simulink model "uav-pid"  (R2020a)
settings: Solver=ode4  StartTime=0.0  StopTime=100  FixedStep=0.25  RelTol=1e-3
libraries: simulink x6
settings Model: Creator=baron  LastModifiedBy=baron

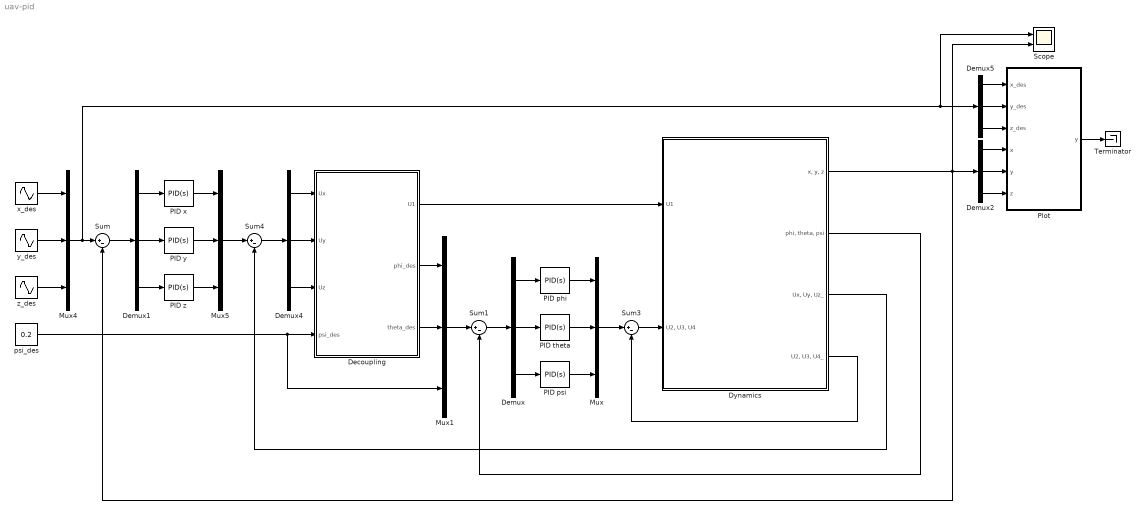
== system uav-pid ==
  Decoupling : MATLAB Function  TreatAsAtomicUnit=on
  Demux{,1..2,4..5} (5 alike) : Demux  Outputs=3
  Dynamics : Subsystem
  Mux{,1,4..5} (4 alike) : Mux  Inputs=3
  PID phi : simulink/Continuous/PID Controller  Controller=PID  Form=Parallel  TimeDomain=Continuous-time  UseExternalTs=off  SampleTime=-1  IntegratorMethod=Forward Euler  FilterMethod=Forward Euler  ControllerParametersSource=internal  P=0.00360663400977862  I=0.000168843771504077  D=0.0189174411465633  UseFilter=on  N=5.45397025421619  TunerSelectOption=Transfer Function Based (PID Tuner App)  InitialConditionSource=internal  InitialConditionForIntegrator=0  InitialConditionForFilter=0  DifferentiatorICPrevScaledInput=0  ExternalReset=none  TrackingMode=off  Kt=1  LimitOutput=off  UpperSaturationLimit=inf  LowerSaturationLimit=-inf  LinearizeAsGain=on  AntiWindupMode=none  Kb=1  POutMin=[]  POutMax=[]  IOutMin=[]  IOutMax=[]  DOutMin=[]  DOutMax=[]  NOutMin=[]  NOutMax=[]  SumOutMin=[]  SumOutMax=[]  SaturationOutMin=[]  SaturationOutMax=[]  PParamMin=[]  PParamMax=[]  IParamMin=[]  IParamMax=[]  DParamMin=[]  DParamMax=[]  NParamMin=[]  NParamMax=[]  KbParamMin=[]  KbParamMax=[]  KtParamMin=[]  KtParamMax=[]  KbOutMin=[]  KbOutMax=[]  KtOutMin=[]  KtOutMax=[]  IntegratorOutMin=[]  IntegratorOutMax=[]  FilterOutMin=[]  FilterOutMax=[]  SumI1OutMin=[]  SumI1OutMax=[]  SumI2OutMin=[]  SumI2OutMax=[]  SumI3OutMin=[]  SumI3OutMax=[]  SumI4OutMin=[]  SumI4OutMax=[]  SumDOutMin=[]  SumDOutMax=[]  DifferentiatorOutMin=[]  DifferentiatorOutMax=[]  FilterDiffOutCoefMin=[]  FilterDiffOutCoefMax=[]  ReciprocalOutMin=[]  ReciprocalOutMax=[]  SumDenOutMin=[]  SumDenOutMax=[]  SumNumOutMin=[]  SumNumOutMax=[]  DivideOutMin=[]  DivideOutMax=[]  UdiffTsProdOutMin=[]  UdiffTsProdOutMax=[]  NTsProdOutMin=[]  NTsProdOutMax=[]  UintegralTsProdOutMin=[]  UintegralTsProdOutMax=[]  UngainTsProdOutMin=[]  UngainTsProdOutMax=[]  IntegratorContinuousStateAttributes=''  IntegratorStateMustResolveToSignalObject=off  IntegratorRTWStateStorageClass=Auto  FilterContinuousStateAttributes=''  FilterStateMustResolveToSignalObject=off  FilterRTWStateStorageClass=Auto  ParallelPVariant=InternalParameters  IdealPVariant=Disabled  IVariant=InternalParameters  DVariant=InternalParameters  IntegratorVariant=Continuous  SatVariant=Disabled  AWVariant=Passthrough  PCopyVariant=Disabled  TRVariant=Disabled  FdbkBlocksVariant=Forward  IdealPFdbkVariant=Disabled  SatFdbkVariant=Disabled  DerivativeFilterVariant=ContFilter  NVariant=InternalParameters  NCopyVariant=Disabled  FilterICVariant=InternalICsFilter  IntegratorICVariant=InternalICs  ExternalResetVariant=Disabled  TRSumVariant=Passthrough  SumFdbkVariant=Disabled  SumVariant=Sum_PID  TsampFilterVariant=InternalTs  TsampNgainVariant=Passthrough  TsampIntegralVariant=Passthrough
  PID psi : simulink/Continuous/PID Controller  Controller=PID  Form=Parallel  TimeDomain=Continuous-time  UseExternalTs=off  SampleTime=-1  IntegratorMethod=Forward Euler  FilterMethod=Forward Euler  ControllerParametersSource=internal  P=0.0016341631960493  I=7.65029876960143e-05  D=0.00857147855904571  UseFilter=on  N=5.45397025421619  TunerSelectOption=Transfer Function Based (PID Tuner App)  InitialConditionSource=internal  InitialConditionForIntegrator=0  InitialConditionForFilter=0  DifferentiatorICPrevScaledInput=0  ExternalReset=none  TrackingMode=off  Kt=1  LimitOutput=off  UpperSaturationLimit=inf  LowerSaturationLimit=-inf  LinearizeAsGain=on  AntiWindupMode=none  Kb=1  POutMin=[]  POutMax=[]  IOutMin=[]  IOutMax=[]  DOutMin=[]  DOutMax=[]  NOutMin=[]  NOutMax=[]  SumOutMin=[]  SumOutMax=[]  SaturationOutMin=[]  SaturationOutMax=[]  PParamMin=[]  PParamMax=[]  IParamMin=[]  IParamMax=[]  DParamMin=[]  DParamMax=[]  NParamMin=[]  NParamMax=[]  KbParamMin=[]  KbParamMax=[]  KtParamMin=[]  KtParamMax=[]  KbOutMin=[]  KbOutMax=[]  KtOutMin=[]  KtOutMax=[]  IntegratorOutMin=[]  IntegratorOutMax=[]  FilterOutMin=[]  FilterOutMax=[]  SumI1OutMin=[]  SumI1OutMax=[]  SumI2OutMin=[]  SumI2OutMax=[]  SumI3OutMin=[]  SumI3OutMax=[]  SumI4OutMin=[]  SumI4OutMax=[]  SumDOutMin=[]  SumDOutMax=[]  DifferentiatorOutMin=[]  DifferentiatorOutMax=[]  FilterDiffOutCoefMin=[]  FilterDiffOutCoefMax=[]  ReciprocalOutMin=[]  ReciprocalOutMax=[]  SumDenOutMin=[]  SumDenOutMax=[]  SumNumOutMin=[]  SumNumOutMax=[]  DivideOutMin=[]  DivideOutMax=[]  UdiffTsProdOutMin=[]  UdiffTsProdOutMax=[]  NTsProdOutMin=[]  NTsProdOutMax=[]  UintegralTsProdOutMin=[]  UintegralTsProdOutMax=[]  UngainTsProdOutMin=[]  UngainTsProdOutMax=[]  IntegratorContinuousStateAttributes=''  IntegratorStateMustResolveToSignalObject=off  IntegratorRTWStateStorageClass=Auto  FilterContinuousStateAttributes=''  FilterStateMustResolveToSignalObject=off  FilterRTWStateStorageClass=Auto  ParallelPVariant=InternalParameters  IdealPVariant=Disabled  IVariant=InternalParameters  DVariant=InternalParameters  IntegratorVariant=Continuous  SatVariant=Disabled  AWVariant=Passthrough  PCopyVariant=Disabled  TRVariant=Disabled  FdbkBlocksVariant=Forward  IdealPFdbkVariant=Disabled  SatFdbkVariant=Disabled  DerivativeFilterVariant=ContFilter  NVariant=InternalParameters  NCopyVariant=Disabled  FilterICVariant=InternalICsFilter  IntegratorICVariant=InternalICs  ExternalResetVariant=Disabled  TRSumVariant=Passthrough  SumFdbkVariant=Disabled  SumVariant=Sum_PID  TsampFilterVariant=InternalTs  TsampNgainVariant=Passthrough  TsampIntegralVariant=Passthrough
  PID theta : simulink/Continuous/PID Controller  Controller=PID  Form=Parallel  TimeDomain=Continuous-time  UseExternalTs=off  SampleTime=-1  IntegratorMethod=Forward Euler  FilterMethod=Forward Euler  ControllerParametersSource=internal  P=0.00360663400977862  I=0.000168843771504077  D=0.0189174411465633  UseFilter=on  N=5.45397025421619  TunerSelectOption=Transfer Function Based (PID Tuner App)  InitialConditionSource=internal  InitialConditionForIntegrator=0  InitialConditionForFilter=0  DifferentiatorICPrevScaledInput=0  ExternalReset=none  TrackingMode=off  Kt=1  LimitOutput=off  UpperSaturationLimit=inf  LowerSaturationLimit=-inf  LinearizeAsGain=on  AntiWindupMode=none  Kb=1  POutMin=[]  POutMax=[]  IOutMin=[]  IOutMax=[]  DOutMin=[]  DOutMax=[]  NOutMin=[]  NOutMax=[]  SumOutMin=[]  SumOutMax=[]  SaturationOutMin=[]  SaturationOutMax=[]  PParamMin=[]  PParamMax=[]  IParamMin=[]  IParamMax=[]  DParamMin=[]  DParamMax=[]  NParamMin=[]  NParamMax=[]  KbParamMin=[]  KbParamMax=[]  KtParamMin=[]  KtParamMax=[]  KbOutMin=[]  KbOutMax=[]  KtOutMin=[]  KtOutMax=[]  IntegratorOutMin=[]  IntegratorOutMax=[]  FilterOutMin=[]  FilterOutMax=[]  SumI1OutMin=[]  SumI1OutMax=[]  SumI2OutMin=[]  SumI2OutMax=[]  SumI3OutMin=[]  SumI3OutMax=[]  SumI4OutMin=[]  SumI4OutMax=[]  SumDOutMin=[]  SumDOutMax=[]  DifferentiatorOutMin=[]  DifferentiatorOutMax=[]  FilterDiffOutCoefMin=[]  FilterDiffOutCoefMax=[]  ReciprocalOutMin=[]  ReciprocalOutMax=[]  SumDenOutMin=[]  SumDenOutMax=[]  SumNumOutMin=[]  SumNumOutMax=[]  DivideOutMin=[]  DivideOutMax=[]  UdiffTsProdOutMin=[]  UdiffTsProdOutMax=[]  NTsProdOutMin=[]  NTsProdOutMax=[]  UintegralTsProdOutMin=[]  UintegralTsProdOutMax=[]  UngainTsProdOutMin=[]  UngainTsProdOutMax=[]  IntegratorContinuousStateAttributes=''  IntegratorStateMustResolveToSignalObject=off  IntegratorRTWStateStorageClass=Auto  FilterContinuousStateAttributes=''  FilterStateMustResolveToSignalObject=off  FilterRTWStateStorageClass=Auto  ParallelPVariant=InternalParameters  IdealPVariant=Disabled  IVariant=InternalParameters  DVariant=InternalParameters  IntegratorVariant=Continuous  SatVariant=Disabled  AWVariant=Passthrough  PCopyVariant=Disabled  TRVariant=Disabled  FdbkBlocksVariant=Forward  IdealPFdbkVariant=Disabled  SatFdbkVariant=Disabled  DerivativeFilterVariant=ContFilter  NVariant=InternalParameters  NCopyVariant=Disabled  FilterICVariant=InternalICsFilter  IntegratorICVariant=InternalICs  ExternalResetVariant=Disabled  TRSumVariant=Passthrough  SumFdbkVariant=Disabled  SumVariant=Sum_PID  TsampFilterVariant=InternalTs  TsampNgainVariant=Passthrough  TsampIntegralVariant=Passthrough
  PID x : simulink/Continuous/PID Controller  Controller=PID  Form=Parallel  TimeDomain=Continuous-time  UseExternalTs=off  SampleTime=-1  IntegratorMethod=Forward Euler  FilterMethod=Forward Euler  ControllerParametersSource=internal  P=0.0902401219497739  I=0.0042245713010184  D=0.473325597056722  UseFilter=on  N=5.45397025421619  TunerSelectOption=Transfer Function Based (PID Tuner App)  InitialConditionSource=internal  InitialConditionForIntegrator=0  InitialConditionForFilter=0  DifferentiatorICPrevScaledInput=0  ExternalReset=none  TrackingMode=off  Kt=1  LimitOutput=off  UpperSaturationLimit=inf  LowerSaturationLimit=-inf  LinearizeAsGain=on  AntiWindupMode=none  Kb=1  POutMin=[]  POutMax=[]  IOutMin=[]  IOutMax=[]  DOutMin=[]  DOutMax=[]  NOutMin=[]  NOutMax=[]  SumOutMin=[]  SumOutMax=[]  SaturationOutMin=[]  SaturationOutMax=[]  PParamMin=[]  PParamMax=[]  IParamMin=[]  IParamMax=[]  DParamMin=[]  DParamMax=[]  NParamMin=[]  NParamMax=[]  KbParamMin=[]  KbParamMax=[]  KtParamMin=[]  KtParamMax=[]  KbOutMin=[]  KbOutMax=[]  KtOutMin=[]  KtOutMax=[]  IntegratorOutMin=[]  IntegratorOutMax=[]  FilterOutMin=[]  FilterOutMax=[]  SumI1OutMin=[]  SumI1OutMax=[]  SumI2OutMin=[]  SumI2OutMax=[]  SumI3OutMin=[]  SumI3OutMax=[]  SumI4OutMin=[]  SumI4OutMax=[]  SumDOutMin=[]  SumDOutMax=[]  DifferentiatorOutMin=[]  DifferentiatorOutMax=[]  FilterDiffOutCoefMin=[]  FilterDiffOutCoefMax=[]  ReciprocalOutMin=[]  ReciprocalOutMax=[]  SumDenOutMin=[]  SumDenOutMax=[]  SumNumOutMin=[]  SumNumOutMax=[]  DivideOutMin=[]  DivideOutMax=[]  UdiffTsProdOutMin=[]  UdiffTsProdOutMax=[]  NTsProdOutMin=[]  NTsProdOutMax=[]  UintegralTsProdOutMin=[]  UintegralTsProdOutMax=[]  UngainTsProdOutMin=[]  UngainTsProdOutMax=[]  IntegratorContinuousStateAttributes=''  IntegratorStateMustResolveToSignalObject=off  IntegratorRTWStateStorageClass=Auto  FilterContinuousStateAttributes=''  FilterStateMustResolveToSignalObject=off  FilterRTWStateStorageClass=Auto  ParallelPVariant=InternalParameters  IdealPVariant=Disabled  IVariant=InternalParameters  DVariant=InternalParameters  IntegratorVariant=Continuous  SatVariant=Disabled  AWVariant=Passthrough  PCopyVariant=Disabled  TRVariant=Disabled  FdbkBlocksVariant=Forward  IdealPFdbkVariant=Disabled  SatFdbkVariant=Disabled  DerivativeFilterVariant=ContFilter  NVariant=InternalParameters  NCopyVariant=Disabled  FilterICVariant=InternalICsFilter  IntegratorICVariant=InternalICs  ExternalResetVariant=Disabled  TRSumVariant=Passthrough  SumFdbkVariant=Disabled  SumVariant=Sum_PID  TsampFilterVariant=InternalTs  TsampNgainVariant=Passthrough  TsampIntegralVariant=Passthrough
  PID y : simulink/Continuous/PID Controller  Controller=PID  Form=Parallel  TimeDomain=Continuous-time  UseExternalTs=off  SampleTime=-1  IntegratorMethod=Forward Euler  FilterMethod=Forward Euler  ControllerParametersSource=internal  P=0.0902401219497739  I=0.0042245713010184  D=0.473325597056722  UseFilter=on  N=5.45397025421619  TunerSelectOption=Transfer Function Based (PID Tuner App)  InitialConditionSource=internal  InitialConditionForIntegrator=0  InitialConditionForFilter=0  DifferentiatorICPrevScaledInput=0  ExternalReset=none  TrackingMode=off  Kt=1  LimitOutput=off  UpperSaturationLimit=inf  LowerSaturationLimit=-inf  LinearizeAsGain=on  AntiWindupMode=none  Kb=1  POutMin=[]  POutMax=[]  IOutMin=[]  IOutMax=[]  DOutMin=[]  DOutMax=[]  NOutMin=[]  NOutMax=[]  SumOutMin=[]  SumOutMax=[]  SaturationOutMin=[]  SaturationOutMax=[]  PParamMin=[]  PParamMax=[]  IParamMin=[]  IParamMax=[]  DParamMin=[]  DParamMax=[]  NParamMin=[]  NParamMax=[]  KbParamMin=[]  KbParamMax=[]  KtParamMin=[]  KtParamMax=[]  KbOutMin=[]  KbOutMax=[]  KtOutMin=[]  KtOutMax=[]  IntegratorOutMin=[]  IntegratorOutMax=[]  FilterOutMin=[]  FilterOutMax=[]  SumI1OutMin=[]  SumI1OutMax=[]  SumI2OutMin=[]  SumI2OutMax=[]  SumI3OutMin=[]  SumI3OutMax=[]  SumI4OutMin=[]  SumI4OutMax=[]  SumDOutMin=[]  SumDOutMax=[]  DifferentiatorOutMin=[]  DifferentiatorOutMax=[]  FilterDiffOutCoefMin=[]  FilterDiffOutCoefMax=[]  ReciprocalOutMin=[]  ReciprocalOutMax=[]  SumDenOutMin=[]  SumDenOutMax=[]  SumNumOutMin=[]  SumNumOutMax=[]  DivideOutMin=[]  DivideOutMax=[]  UdiffTsProdOutMin=[]  UdiffTsProdOutMax=[]  NTsProdOutMin=[]  NTsProdOutMax=[]  UintegralTsProdOutMin=[]  UintegralTsProdOutMax=[]  UngainTsProdOutMin=[]  UngainTsProdOutMax=[]  IntegratorContinuousStateAttributes=''  IntegratorStateMustResolveToSignalObject=off  IntegratorRTWStateStorageClass=Auto  FilterContinuousStateAttributes=''  FilterStateMustResolveToSignalObject=off  FilterRTWStateStorageClass=Auto  ParallelPVariant=InternalParameters  IdealPVariant=Disabled  IVariant=InternalParameters  DVariant=InternalParameters  IntegratorVariant=Continuous  SatVariant=Disabled  AWVariant=Passthrough  PCopyVariant=Disabled  TRVariant=Disabled  FdbkBlocksVariant=Forward  IdealPFdbkVariant=Disabled  SatFdbkVariant=Disabled  DerivativeFilterVariant=ContFilter  NVariant=InternalParameters  NCopyVariant=Disabled  FilterICVariant=InternalICsFilter  IntegratorICVariant=InternalICs  ExternalResetVariant=Disabled  TRSumVariant=Passthrough  SumFdbkVariant=Disabled  SumVariant=Sum_PID  TsampFilterVariant=InternalTs  TsampNgainVariant=Passthrough  TsampIntegralVariant=Passthrough
  PID z : simulink/Continuous/PID Controller  Controller=PID  Form=Parallel  TimeDomain=Continuous-time  UseExternalTs=off  SampleTime=-1  IntegratorMethod=Forward Euler  FilterMethod=Forward Euler  ControllerParametersSource=internal  P=0.0902401219497739  I=0.0042245713010184  D=0.473325597056722  UseFilter=on  N=5.45397025421619  TunerSelectOption=Transfer Function Based (PID Tuner App)  InitialConditionSource=internal  InitialConditionForIntegrator=0  InitialConditionForFilter=0  DifferentiatorICPrevScaledInput=0  ExternalReset=none  TrackingMode=off  Kt=1  LimitOutput=off  UpperSaturationLimit=inf  LowerSaturationLimit=-inf  LinearizeAsGain=on  AntiWindupMode=none  Kb=1  POutMin=[]  POutMax=[]  IOutMin=[]  IOutMax=[]  DOutMin=[]  DOutMax=[]  NOutMin=[]  NOutMax=[]  SumOutMin=[]  SumOutMax=[]  SaturationOutMin=[]  SaturationOutMax=[]  PParamMin=[]  PParamMax=[]  IParamMin=[]  IParamMax=[]  DParamMin=[]  DParamMax=[]  NParamMin=[]  NParamMax=[]  KbParamMin=[]  KbParamMax=[]  KtParamMin=[]  KtParamMax=[]  KbOutMin=[]  KbOutMax=[]  KtOutMin=[]  KtOutMax=[]  IntegratorOutMin=[]  IntegratorOutMax=[]  FilterOutMin=[]  FilterOutMax=[]  SumI1OutMin=[]  SumI1OutMax=[]  SumI2OutMin=[]  SumI2OutMax=[]  SumI3OutMin=[]  SumI3OutMax=[]  SumI4OutMin=[]  SumI4OutMax=[]  SumDOutMin=[]  SumDOutMax=[]  DifferentiatorOutMin=[]  DifferentiatorOutMax=[]  FilterDiffOutCoefMin=[]  FilterDiffOutCoefMax=[]  ReciprocalOutMin=[]  ReciprocalOutMax=[]  SumDenOutMin=[]  SumDenOutMax=[]  SumNumOutMin=[]  SumNumOutMax=[]  DivideOutMin=[]  DivideOutMax=[]  UdiffTsProdOutMin=[]  UdiffTsProdOutMax=[]  NTsProdOutMin=[]  NTsProdOutMax=[]  UintegralTsProdOutMin=[]  UintegralTsProdOutMax=[]  UngainTsProdOutMin=[]  UngainTsProdOutMax=[]  IntegratorContinuousStateAttributes=''  IntegratorStateMustResolveToSignalObject=off  IntegratorRTWStateStorageClass=Auto  FilterContinuousStateAttributes=''  FilterStateMustResolveToSignalObject=off  FilterRTWStateStorageClass=Auto  ParallelPVariant=InternalParameters  IdealPVariant=Disabled  IVariant=InternalParameters  DVariant=InternalParameters  IntegratorVariant=Continuous  SatVariant=Disabled  AWVariant=Passthrough  PCopyVariant=Disabled  TRVariant=Disabled  FdbkBlocksVariant=Forward  IdealPFdbkVariant=Disabled  SatFdbkVariant=Disabled  DerivativeFilterVariant=ContFilter  NVariant=InternalParameters  NCopyVariant=Disabled  FilterICVariant=InternalICsFilter  IntegratorICVariant=InternalICs  ExternalResetVariant=Disabled  TRSumVariant=Passthrough  SumFdbkVariant=Disabled  SumVariant=Sum_PID  TsampFilterVariant=InternalTs  TsampNgainVariant=Passthrough  TsampIntegralVariant=Passthrough
  Plot : MATLAB Function  TreatAsAtomicUnit=on
  Scope : Scope  NumInputPorts=2
  Sum{,1,3..4} (4 alike) : Sum  Inputs=|+-
  Terminator : Terminator
  psi_des : Constant  Value=0.2
  x_des : Sin  Amplitude=8  Bias=1  Frequency=0.1  SampleTime=0
  y_des : Sin  Amplitude=8  Bias=-8  Frequency=0.1  Phase=pi/2  SampleTime=0
  z_des : Sin  Amplitude=3  Bias=6  Frequency=0.2  Phase=3*pi/2  SampleTime=0
  wires:
  Decoupling/1(U1) -> Dynamics/1(U1)
  y_des/1 -> Mux4/2
  x_des/1 -> Mux4/1
  Decoupling/2(phi_des) -> Mux1/1
  Decoupling/3(theta_des) -> Mux1/2
  Mux4/1 -> Sum/1, Scope/1, Demux5/1
  Mux1/1 -> Sum1/1
  Dynamics/1("x, y, z") -> Scope/2, Demux2/1, Sum/2
  Dynamics/2("phi, theta, psi") -> Sum1/2
  Demux/2 -> PID theta/1
  Demux/3 -> PID psi/1
  Demux/1 -> PID phi/1
  Sum1/1 -> Demux/1
  Demux1/1 -> PID x/1
  Demux1/2 -> PID y/1
  Demux1/3 -> PID z/1
  Sum/1 -> Demux1/1
  psi_des/1 -> Decoupling/4(psi_des), Mux1/3
  Demux2/3 -> Plot/6(z)
  Demux2/2 -> Plot/5("y ")
  Demux2/1 -> Plot/4(x)
  Plot/1(y) -> Terminator/1
  PID psi/1 -> Mux/3
  PID theta/1 -> Mux/2
  PID phi/1 -> Mux/1
  Mux/1 -> Sum3/1
  Sum3/1 -> Dynamics/2("U2, U3, U4")
  Dynamics/4("U2, U3, U4_") -> Sum3/2
  PID x/1 -> Mux5/1
  PID y/1 -> Mux5/2
  PID z/1 -> Mux5/3
  Demux4/1 -> Decoupling/1(Ux)
  Demux4/2 -> Decoupling/2(Uy)
  Demux4/3 -> Decoupling/3(Uz)
  Sum4/1 -> Demux4/1
  Mux5/1 -> Sum4/1
  Dynamics/3("Ux, Uy, Uz_") -> Sum4/2
  Demux5/1 -> Plot/1(x_des)
  Demux5/2 -> Plot/2(y_des)
  Demux5/3 -> Plot/3(z_des)
  z_des/1 -> Mux4/3

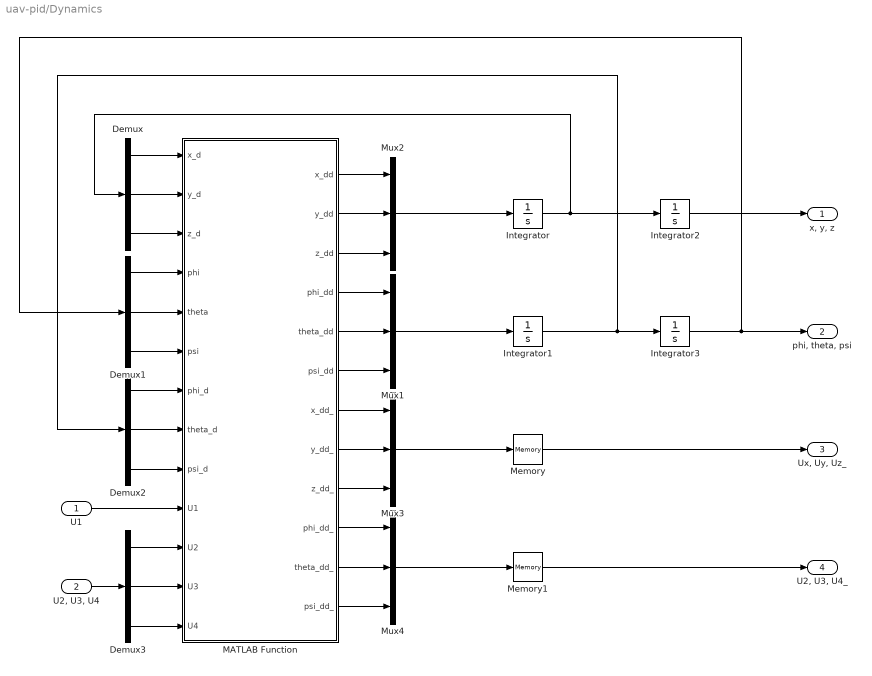
== system uav-pid/Dynamics ==
  U1 : Inport
  "U2, U3, U4" : Inport  Port=2
  Demux{,1..3} (4 alike) : Demux  Outputs=3
  Integrator{,1..3} (4 alike) : Integrator
  MATLAB Function : MATLAB Function  TreatAsAtomicUnit=on
  Memory : Memory
  Memory1 : Memory
  Mux{1..4} (4 alike) : Mux  Inputs=3
  "x, y, z" : Outport
  "phi, theta, psi" : Outport  Port=2
  "Ux, Uy, Uz_" : Outport  Port=3
  "U2, U3, U4_" : Outport  Port=4
  wires:
  U1/1 -> MATLAB Function/10(U1)
  Demux3/2 -> MATLAB Function/12(U3)
  Demux3/1 -> MATLAB Function/11(U2)
  Demux3/3 -> MATLAB Function/13(U4)
  MATLAB Function/3(z_dd) -> Mux2/3
  MATLAB Function/4(phi_dd) -> Mux1/1
  MATLAB Function/5(theta_dd) -> Mux1/2
  MATLAB Function/6(psi_dd) -> Mux1/3
  Mux2/1 -> Integrator/1
  Mux1/1 -> Integrator1/1
  Integrator/1 -> Integrator2/1, Demux/1
  Integrator1/1 -> Integrator3/1, Demux2/1
  Demux/1 -> MATLAB Function/1(x_d)
  Demux/2 -> MATLAB Function/2(y_d)
  Demux/3 -> MATLAB Function/3(z_d)
  Demux1/1 -> MATLAB Function/4(phi)
  Demux1/2 -> MATLAB Function/5(theta)
  Demux1/3 -> MATLAB Function/6(psi)
  Demux2/1 -> MATLAB Function/7(phi_d)
  Demux2/2 -> MATLAB Function/8(theta_d)
  Demux2/3 -> MATLAB Function/9(psi_d)
  Integrator3/1 -> "phi, theta, psi"/1, Demux1/1
  Integrator2/1 -> "x, y, z"/1
  MATLAB Function/1(x_dd) -> Mux2/1
  MATLAB Function/2(y_dd) -> Mux2/2
  MATLAB Function/7(x_dd_) -> Mux3/1
  MATLAB Function/8(y_dd_) -> Mux3/2
  MATLAB Function/9(z_dd_) -> Mux3/3
  MATLAB Function/10(phi_dd_) -> Mux4/1
  MATLAB Function/11(theta_dd_) -> Mux4/2
  MATLAB Function/12(psi_dd_) -> Mux4/3
  Mux3/1 -> Memory/1
  Memory/1 -> "Ux, Uy, Uz_"/1
  Mux4/1 -> Memory1/1
  Memory1/1 -> "U2, U3, U4_"/1
  "U2, U3, U4"/1 -> Demux3/1

== matlab function uav-pid/Decoupling ==
  data: U1 output; phi_des output; Ux input; theta_des output; Uy input; Uz input; psi_des input
function [U1, phi_des, theta_des] = fcn(Ux, Uy, Uz, psi_des)
U1 = sqrt(Ux^2 + Uy^2 + Uz^2);
theta_des = atan((Ux*cos(psi_des) + Uy*sin(psi_des))/(Uz));
phi_des = atan(cos(theta_des)*(Ux*sin(psi_des) - Uy*cos(psi_des))/(Uz));

== matlab function uav-pid/Dynamics/MATLAB Function ==
  data: x_dd output; x_d input; y_d input; z_d input; phi input; theta input; psi input; phi_d input; theta_d input; psi_d input; y_dd output; U1 input; U2 input; U3 input; U4 input; z_dd output; phi_dd output; theta_dd output; psi_dd output; x_dd_ output; y_dd_ output; z_dd_ output; phi_dd_ output; theta_dd_ output; psi_dd_ output
function [x_dd, y_dd, z_dd, phi_dd, theta_dd, psi_dd, x_dd_, y_dd_, z_dd_, phi_dd_, theta_dd_, psi_dd_]= fcn(x_d, y_d, z_d, phi, theta, psi, phi_d, theta_d, psi_d, U1, U2, U3, U4)
    m = 0.486;
    g = 9.810;
    l = 0.250;
    Ixx = 4.856e-3;
    Iyy = 4.856e-3;
    Izz = 8.801e-3;
    cdx = 5.560e-4;
    cdy = 5.560e-4;
    cdz = 6.350e-4;
x_dd = (-1/m)*cdx*x_d + (1/m)*(cos(phi)*cos(psi)*sin(theta) + sin(phi)*sin(psi))*U1;
y_dd = (-1/m)*cdy*y_d + (1/m)*(cos(phi)*sin(psi)*sin(theta) - sin(phi)*cos(psi))*U1;
z_dd = (-1/m)*cdz*z_d - g + (1/m)*(cos(phi)*cos(theta))*U1;
phi_dd = ((Iyy - Izz)/Ixx)*theta_d*psi_d + (l/Ixx)*U2;
theta_dd = ((Izz - Ixx)/Iyy)*phi_d*psi_d + (l/Iyy)*U3;
psi_dd = ((Ixx - Iyy)/Izz)*phi_d*theta_d + (1/Izz)*U4;
x_dd_ = ((-1/m)*cdx*x_d)/(1/m);
y_dd_ = ((-1/m)*cdy*y_d)/(1/m);
z_dd_ = ((-1/m)*cdz*z_d - g)/(1/m);
phi_dd_ = (((Iyy - Izz)/Ixx)*theta_d*psi_d)/(l/Ixx);
theta_dd_ = (((Izz - Ixx)/Iyy)*phi_d*psi_d)/(l/Iyy);
psi_dd_ = (((Ixx - Iyy)/Izz)*phi_d*theta_d)/(1/Izz);

== matlab function uav-pid/Plot ==
  data: x_des input; y_des input; z_des input; x input; y output; y input; z input
function y = fcn(x_des, y_des, z_des, x, y, z)
    grid on;
    plot3(x, y, z, 'b.');
    hold on;
    plot3(x_des, y_des, z_des, 'r.');
y = 0;
